simulink model "pe_electric_engine_dyno"  (R2017b)
settings: Solver=FixedStepDiscrete  StartTime=0.0  StopTime=0.8  FixedStep=Ts  RelTol=1e-3  EnableMultiTasking=on
PreLoadFcn:
  | pe_electric_engine_dyno_data;
values from neighbouring files (symbols this model uses):
  ce = 25    [pe_electric_engine_dyno_data.m]
  fn = 60    [pe_electric_engine_dyno_data.m]
  Ibase = Pn/(1.5*Vbase)    [pe_electric_engine_dyno_data.m]
  Ld = 0.00024368    [pe_electric_engine_dyno_data.m]
  Lm = 2.717    [pe_electric_engine_dyno_data.m]
  Lq = 0.00029758    [pe_electric_engine_dyno_data.m]
  p = 8    [pe_electric_engine_dyno_data.m]
  p2 = 2    [pe_electric_engine_dyno_data.m]
  psim = 0.04366    [pe_electric_engine_dyno_data.m]
  Ts = 5e-6    (= 5e-06)    [init_model_Ffwd.m]    (also in pe_electric_engine_dyno_data.m = 1e-05)
  Tsc = 1/(fsw2*5)    (= 0.0001)    [pe_electric_engine_dyno_data.m]
  Xls = Lls*Zbase    [pe_electric_engine_dyno_data.m]
undefined symbols (not defined in the file or in its folder): pe, sigbuilder_block, VDC_VECT
libraries: nesl_utility x22, fl_lib x15, pe_lib x12, peTransforms x2, peAsmFieldOrientedControl x1, peGeneralControl x1, pePmsmCurrentController x1, simulink x1, pePmsmCurrentReferenceGen x1, pePmsmTorqueEstimator x1, pePwmGeneratorTwoLevel x1
Description:
  | Electric Engine Dyno
  | 
  | This example shows how to model an electric vehicle dynamometer test.
  | The test environment contains an asynchronous machine (ASM) and an
  | interior permanent magnet synchronous machine (IPMSM) connected back-
  | to-back through a mechanical shaft. Both machines are fed by high-
  | voltage batteries through controlled three-phase converters. The 164 kW
  | ASM produces the load torque. The 35 kW IPMSM is the electric machine
  | under test. The Control Machine Under Test (IPMSM) subsystem controls the
  | torque of the IPMSM. The controller includes a multi-rate PI-based
  | control structure. The rate of the open-loop torque control is slower
  | than the rate of the closed-loop current control. The task scheduling
  | for the controller is implemented as a Stateflow(TM) state machine. The
  | Control Load Machine (ASM) subsystem uses a single rate to control the
  | speed of the ASM. The Visualization subsystem contains scopes that
  | allow you to see the simulation results.
settings Model: Creator=The MathWorks, Inc.  LastModifiedBy=The MathWorks, Inc.
settings OptimizationCC: LifeSpan=inf
settings DebuggingCC: UnderspecifiedInitializationDetection=Classic  MergeDetectMultiDrivingBlocksExec=none  SFUnexpectedBacktrackingDiag=warning  SFNoUnconditionalDefaultTransitionDiag=warning  SFExecutionAtInitializationDiag=none
settings CodeAppCC: StateflowObjectComments=on
settings GRTTargetCC: TargetLangStandard=C89/C90 (ANSI)  GeneratePreprocessorConditionals=Disable all
settings ConfigComp: CovMetricSettings=dw  CovHtmlReporting=on  CovSaveCumulativeToWorkspaceVar=on  CovSaveSingleToWorkspaceVar=on  CovExternalEMLEnable=off
settings SimscapeCC: SimscapeLogType=all  SimscapeLogSimulationStatistics=on  SimscapeLogName=simlog_pe_electric_engine_dyno  SimscapeLogLimitData=off

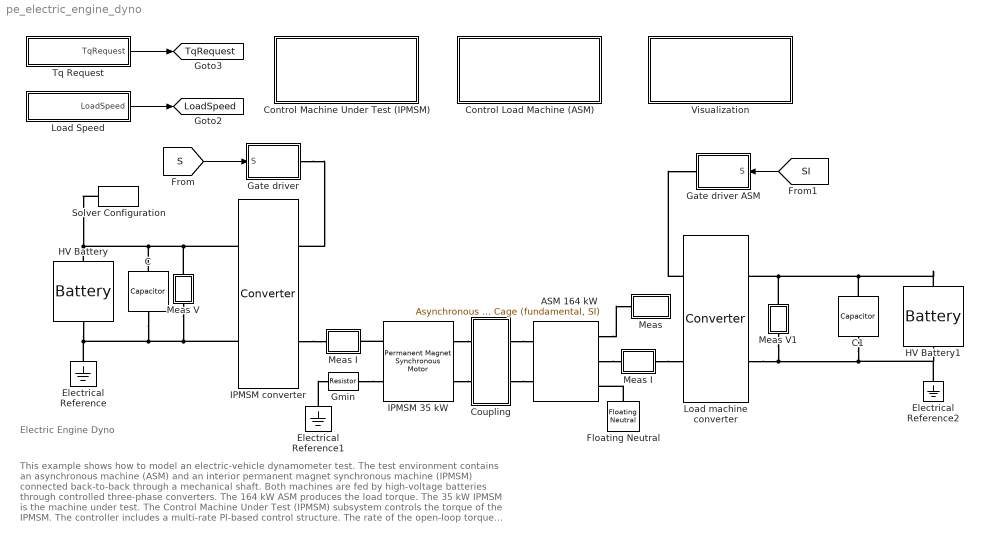
== system pe_electric_engine_dyno ==
  note: This example shows how to model an electric-vehicle dynamometer test. The test environment contains an asynchronous machine (ASM) and an interior permanent magnet synchronous machine (IPMSM) connected back-to-back through a mechanical shaft. Both machines are fed by high-voltage batteries through controlled three-phase converters. The 164 kW ASM produces the load torque. The 35 kW IPMSM is the machine under test. The Control Machine Under Test (IPMSM) subsystem controls the torque of the IPMSM. The controller includes a multi-rate PI-based control structure. The rate of the open-loop torque control is slower than the rate of the closed-loop current control. The task scheduling for the controller is implemented as a Stateflow(TM) state machine. The Control Load Machine (ASM) subsystem uses a single rate to control the speed of the ASM. The Visualization subsystem contains scopes that allow you to see the simulation results.
      | Edit associated parameterization script.
      | Explore simulation results using sscexplore .
      | Learn more about this example.
  note: Electric Engine Dyno
  ASM 164 kW : pe_lib/Machines/Asynchronous Machine (Squirrel Cage)/Asynchronous Machine Squirrel Cage (fundamental, SI)  SRated=Pn V*A  VRated=Vn V  FRated=fn Hz  nPolePairs=p2  Rs=Rss Ohm  Xls=Xls Ohm  Rrd=Rrr Ohm  Xlrd=Xlr Ohm  Xm=Xm Ohm  X0=Xls Ohm  angular_position0=0 deg  psids0=0 Wb  psiqs0=0 Wb  psi0s0=0 Wb  psidr0=0 Wb  psiqr0=0 Wb  connection_option=int32(pe.Connection.delta)
      settings: SourceProductName=Simscape Power Systems  SourceProductBaseCode=PS
  C : fl_lib/Electrical/Electrical Elements/Capacitor  c=Cdc F  r=1e-6 Ohm  g=0 1/Ohm  i_specify=off  i_priority=None  i=0 A  i_nominal_specify=off  i_nominal_unit=A  i_nominal_value=1  v_specify=off  v_priority=None  v=0 V  v_nominal_specify=off  v_nominal_unit=V  v_nominal_value=1  vc_specify=off  vc_priority=High  vc=0 V  vc_nominal_specify=off  vc_nominal_unit=V  vc_nominal_value=1
      settings: SourceProductName=Foundation Library
  C1 : fl_lib/Electrical/Electrical Elements/Capacitor  c=Cdc F  r=1e-6 Ohm  g=0 1/Ohm  i_specify=off  i_priority=None  i=0 A  i_nominal_specify=off  i_nominal_unit=A  i_nominal_value=1  v_specify=off  v_priority=None  v=0 V  v_nominal_specify=off  v_nominal_unit=V  v_nominal_value=1  vc_specify=off  vc_priority=High  vc=0 V  vc_nominal_specify=off  vc_nominal_unit=V  vc_nominal_value=1
      settings: SourceProductName=Foundation Library
  Control Load Machine (ASM) : Subsystem
  Control Machine Under Test (IPMSM) : Subsystem
  Coupling : Subsystem
  Electrical Reference : fl_lib/Electrical/Electrical Elements/Electrical Reference
      settings: SourceProductName=Foundation Library
  Electrical Reference1 : fl_lib/Electrical/Electrical Elements/Electrical Reference
      settings: SourceProductName=Foundation Library
  Electrical Reference2 : fl_lib/Electrical/Electrical Elements/Electrical Reference
      settings: SourceProductName=Foundation Library
  Floating Neutral : pe_lib/Connections/Floating Neutral
      settings: SourceProductName=Simscape Power Systems  SourceProductBaseCode=PS
  Gate driver : Subsystem
  Gate driver ASM : Subsystem
  Gmin : fl_lib/Electrical/Electrical Elements/Resistor  R=1e9 Ohm  i_specify=off  i_priority=High  i=0 A  i_nominal_specify=off  i_nominal_unit=A  i_nominal_value=1  v_specify=off  v_priority=High  v=0 V  v_nominal_specify=off  v_nominal_unit=V  v_nominal_value=1
      settings: SourceProductName=Foundation Library
  HV Battery : pe_lib/Sources/Battery  Vnom=Vnom V  R1=0.001 Ohm  prm_AH=2  AH=10000 hr*A  V1=V1 V  AH1=3000 hr*A  prm_R2=1  R2=2000 Ohm  prm_fade=1  N_fade=100  AH_fade=45 hr*A  R1_fade=2.02 Ohm  V1_fade=10.35 V  i_specify=off  i_priority=None  i=0 A  i_nominal_specify=off  i_nominal_unit=A  i_nominal_value=1  v_specify=off  v_priority=None  v=0 V  v_nominal_specify=off  v_nominal_unit=V  v_nominal_value=1  charge_specify=on  charge_priority=High  charge=8000 hr*A  charge_nominal_specify=off  charge_nominal_unit=hr*A  charge_nominal_value=1  num_cycles_specify=off  num_cycles_priority=High  num_cycles=0  num_cycles_nominal_specify=off  num_cycles_nominal_unit=1  num_cycles_nominal_value=1  thermal_mass=30000 J/K  Tmeas=298.15 K  Vnom_T2=12 V  R1_T2=2.2 Ohm  V1_T2=11.4 V  R2_T2=2200 Ohm  Tmeas2=273.15 K  temperature_specify=off  temperature_priority=High  temperature=298.15 K  temperature_nominal_specify=off  temperature_nominal_unit=K  temperature_nominal_value=1
      settings: SourceProductName=Simscape Power Systems  SourceProductBaseCode=PS
  HV Battery1 : pe_lib/Sources/Battery  Vnom=775 V  R1=0.001 Ohm  prm_AH=2  AH=25000 hr*A  V1=750 V  AH1=20000 hr*A  prm_R2=1  R2=2000 Ohm  prm_fade=1  N_fade=100  AH_fade=45 hr*A  R1_fade=2.02 Ohm  V1_fade=10.35 V  i_specify=off  i_priority=None  i=0 A  i_nominal_specify=off  i_nominal_unit=A  i_nominal_value=1  v_specify=off  v_priority=None  v=0 V  v_nominal_specify=off  v_nominal_unit=V  v_nominal_value=1  charge_specify=on  charge_priority=High  charge=20000 hr*A  charge_nominal_specify=off  charge_nominal_unit=hr*A  charge_nominal_value=1  num_cycles_specify=off  num_cycles_priority=High  num_cycles=0  num_cycles_nominal_specify=off  num_cycles_nominal_unit=1  num_cycles_nominal_value=1  thermal_mass=30000 J/K  Tmeas=298.15 K  Vnom_T2=12 V  R1_T2=2.2 Ohm  V1_T2=11.4 V  R2_T2=2200 Ohm  Tmeas2=273.15 K  temperature_specify=off  temperature_priority=High  temperature=298.15 K  temperature_nominal_specify=off  temperature_nominal_unit=K  temperature_nominal_value=1
      settings: SourceProductName=Simscape Power Systems  SourceProductBaseCode=PS
  IPMSM 35 kW : pe_lib/Machines/Permanent Magnet Rotor/Permanent Magnet Synchronous Motor  nPolePairs=p  pmflux_param=1  pm_flux_linkage=psim Wb  torque_constant=0.18 N*m/A  back_emf_constant=0.18 V/(rad/s)  stator_param=1  Ld=Ld H  Lq=Lq H  L0=L0 H  Ls=0.0002 H  Lm=0.00002 H  Ms=0.00002 H  Rs=Rs Ohm  initial_currents=[0, 0, 0] A  axes_param=1  angular_position0=0 rad  rotor_offset=- pi / 2 rad  shift_3ph=[nan, nan, nan] rad  sqrt2OverSqrt3=nan  oneOverSqrt2=nan  twoPiOver3=nan  Lmin=1e-9 H
      settings: SourceProductName=Simscape Power Systems  SourceProductBaseCode=PS
  IPMSM converter : pe_lib/Semiconductors/Converter  device_type=3  Vf=0.8 V  Ron=0.001 Ohm  Rds=0.001 Ohm  Goff=1e-5 1/Ohm  Vth=0.5 V  Vgt=1 V  Vgt_off=-1 V  Ih=1 A  diode_param=2  diode_Vf=0.8 V  diode_Ron=0.001 Ohm  diode_Goff=1e-5 1/Ohm  diode_C=50 nF  diode_iRM=-235 A  diode_iF=300 A  diode_idot=-50 A/us  diode_trr_param=1  diode_trr_factor=3  diode_trr=15 us  diode_Qrr=1.5e+3 s*uA  snubber_type=0  Rs=0.1 Ohm  Cs=1e-7 F
      settings: SourceProductName=Simscape Power Systems  SourceProductBaseCode=PS
  Load Speed : Subsystem  Tag=STV Subsys  LoadFcn=sigbuilder_block('load');  StartFcn=sigbuilder_block('start');  StopFcn=sigbuilder_block('stop');  ClipboardFcn=sigbuilder_block('clipboard');  mask(Sigbuilder block){tuvar=[0:10]}
      mask help: Simulink:masks:SigbuilderBlock_MD
      mask init:
      | if ~strcmp(get_param(bdroot(gcbh),'SimulationStatus'),'stopped') tuvar = sigbuilder_block('maskInit'); end
      settings: CopyFcn=sigbuilder_block('copy');  DeleteFcn=sigbuilder_block('delete');  ModelCloseFcn=sigbuilder_block('modelClose');  PreSaveFcn=sigbuilder_block('preSave');  PauseFcn=sigbuilder_block('pause');  ContinueFcn=sigbuilder_block('continue');  NameChangeFcn=sigbuilder_block('namechange');  OpenFcn=sigbuilder_block('open',[324 245.25 633.75 283.5 ]);  CloseFcn=sigbuilder_block('close');
      mask Display: plot(0, 0, 100, 100,[2, 2, 32, 32, 2], [68, 8, 8, 68, 68],[32, 2], [38, 38], [32, 19, 2],[53, 60, 44], [32, 17, 17, 2],[16, 16, 31, 31]);txt = getActiveGroup(gcbh);text(2, 100, txt,'verticalAlignment', 'top');
  Load machine converter : pe_lib/Semiconductors/Converter  device_type=3  Vf=0.8 V  Ron=0.001 Ohm  Rds=0.001 Ohm  Goff=1e-5 1/Ohm  Vth=0.5 V  Vgt=1 V  Vgt_off=-1 V  Ih=1 A  diode_param=2  diode_Vf=0.8 V  diode_Ron=0.001 Ohm  diode_Goff=1e-5 1/Ohm  diode_C=50 nF  diode_iRM=-235 A  diode_iF=300 A  diode_idot=-50 A/us  diode_trr_param=1  diode_trr_factor=3  diode_trr=15 us  diode_Qrr=1.5e+3 s*uA  snubber_type=0  Rs=0.1 Ohm  Cs=1e-7 F
      settings: SourceProductName=Simscape Power Systems  SourceProductBaseCode=PS
  Meas : Subsystem
  Meas I : Subsystem
  "Meas I " : Subsystem
  Meas V : Subsystem
  Meas V1 : Subsystem
  Solver Configuration : nesl_utility/Solver Configuration  PhysicalDomain=network_engine_domain  SubClassName=solver  LeftPortType=input  RightPortType=generic  Accelerate=off  Tones=[]  Harmonics=[]  SimulateNoise=off  Profile=off  UseLocalSampling=off  EnableSwitchedLinearOptims=on  FrequencyDomain=off  UseCCode=off  RelTol=0.001  AbsTol=1e-06  MinStep=1e-09  ToWorkspace=off  RevertToSquareIcSolve=off  NumHomotopyIterations=100  PhasorMode=off  PhasorModeNumHarmonics=1  DoDC=off  ResidualTolerance=1e-9  UseLocalSolver=on  LocalSolverChoice=NE_BACKWARD_EULER_ADVANCER  LocalSolverSampleTime=Ts  DoFixedCost=on  MaxNonlinIter=4  MaxModeIter=2  LinearAlgebra=Sparse  DelaysMemoryBudget=1024  AutomaticFiltering=on  FilteringTimeConstant=0.001
  Tq Request : Subsystem  Tag=STV Subsys  LoadFcn=sigbuilder_block('load');  StartFcn=sigbuilder_block('start');  StopFcn=sigbuilder_block('stop');  ClipboardFcn=sigbuilder_block('clipboard');  mask(Sigbuilder block){tuvar=[0:10]}
      mask help: Simulink:masks:SigbuilderBlock_MD
      mask init:
      | if ~strcmp(get_param(bdroot(gcbh),'SimulationStatus'),'stopped') tuvar = sigbuilder_block('maskInit'); end
      settings: CopyFcn=sigbuilder_block('copy');  DeleteFcn=sigbuilder_block('delete');  ModelCloseFcn=sigbuilder_block('modelClose');  PreSaveFcn=sigbuilder_block('preSave');  PauseFcn=sigbuilder_block('pause');  ContinueFcn=sigbuilder_block('continue');  NameChangeFcn=sigbuilder_block('namechange');  OpenFcn=sigbuilder_block('open',[1556.25 287.25 486.75 260.25 ]);  CloseFcn=sigbuilder_block('close');
      mask Display: plot(0, 0, 100, 100,[2, 2, 32, 32, 2], [68, 8, 8, 68, 68],[32, 2], [38, 38], [32, 19, 2],[53, 60, 44], [32, 17, 17, 2],[16, 16, 31, 31]);txt = getActiveGroup(gcbh);text(2, 100, txt,'verticalAlignment', 'top');
  Visualization : Subsystem
  tag scope: LoadSpeed=global, TqRequest=global
  wires:
  [S] -> Gate driver/1(S)
  [SI] -> Gate driver ASM/1(S)
  Tq Request/1(TqRequest) -> [TqRequest]
  Load Speed/1(LoadSpeed) -> [LoadSpeed]
  connections:
  IPMSM converter/RConn2 -- Meas V/RConn1 -- HV Battery/RConn1 -- Electrical Reference/LConn1 -- C/RConn1
  IPMSM converter/RConn1 -- Meas V/LConn1 -- HV Battery/LConn1 -- Solver Configuration/RConn1 -- C/LConn1
  Electrical Reference1/LConn1 -- Gmin/LConn1
  Gate driver/RConn1 -- IPMSM converter/LConn1
  Floating Neutral/LConn1 -- ASM 164 kW/RConn3
  HV Battery1/LConn1 -- C1/LConn1 -- Load machine converter/RConn1 -- Meas V1/LConn1
  Load machine converter/RConn2 -- Meas V1/RConn1 -- Electrical Reference2/LConn1 -- HV Battery1/RConn1 -- C1/RConn1
  IPMSM 35 kW/RConn2 -- Coupling/LConn2
  Coupling/RConn2 -- ASM 164 kW/LConn2
  IPMSM 35 kW/RConn1 -- Coupling/LConn1
  IPMSM converter/LConn2 -- Meas I/LConn1
  IPMSM 35 kW/LConn1 -- Meas I/RConn1
  Coupling/RConn1 -- ASM 164 kW/LConn1
  Gmin/RConn1 -- IPMSM 35 kW/LConn2
  ASM 164 kW/RConn2 -- "Meas I "/RConn1
  "Meas I "/LConn1 -- Load machine converter/LConn2
  ASM 164 kW/RConn1 -- Meas/LConn1
  Load machine converter/LConn1 -- Gate driver ASM/RConn1

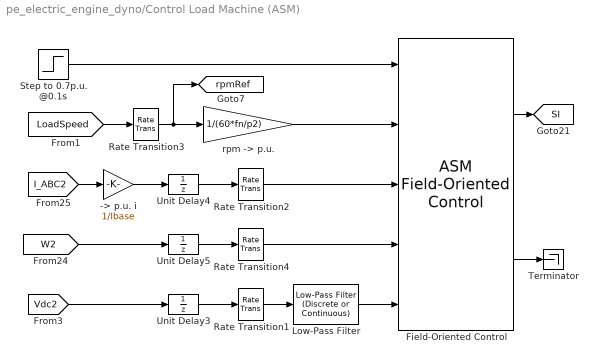
== system pe_electric_engine_dyno/Control Load Machine (ASM) ==
  -> p.u. i : Gain  Gain=1/Ibase
  Field-Oriented Control : peAsmFieldOrientedControl/ASM Field-Oriented Control  Vn=Vn  fn=fn  Rr=Rr  Llr=Llr  Lm=Lm  Tc=1e-4  Vdc_on=400  Ts=Ts  Tsc=Tsc  Kp_imr=Kp_imr  Ki_imr=Ki_imr  Kaw_imr=1000  Kp_wr=Kp_wr  Ki_wr=Ki_wr  Kaw_wr=1000  id_max=2  iq_max=2  AxisAlignment=Q-axis  Kp_id=Kp_ids  Ki_id=Ki_ids  Kaw_id=1000  Kp_iq=Kp_iqs  Ki_iq=Ki_iqs  Kaw_iq=1000  AxisPrio=D-Q equivalence  CPWMMode=SPWM: sinusoidal PWM  fsw=fsw2
      settings: SamplingMode=Natural
  Low-Pass Filter : peGeneralControl/Low-Pass Filter (Discrete or Continuous)  K=1  T=1e-3  B=inf  A=-inf  Ts=Tsc
  Rate Transition{1..4} (4 alike) : RateTransition  OutPortSampleTime=Tsc
  Step to 0.7p.u. @0.1s : Step  Time=0.1  After=0.7*1/Lm  SampleTime=Tsc
  Terminator : Terminator
  Unit Delay3 : UnitDelay  SampleTime=Ts
  Unit Delay4 : UnitDelay  SampleTime=Ts
  Unit Delay5 : UnitDelay  SampleTime=Ts
  "rpm -> p.u." : Gain  Gain=1/(60*fn/p2)
  tag scope: SI=global, rpmRef=global
  wires:
  [LoadSpeed] -> Rate Transition3/1
  Field-Oriented Control/1 -> [SI]
  Unit Delay5/1 -> Rate Transition4/1
  [Vdc2] -> Unit Delay3/1
  Rate Transition2/1 -> Field-Oriented Control/3
  Low-Pass Filter/1 -> Field-Oriented Control/5
  Rate Transition1/1 -> Low-Pass Filter/1
  [W2] -> Unit Delay5/1
  Rate Transition4/1 -> Field-Oriented Control/4
  Unit Delay4/1 -> Rate Transition2/1
  Unit Delay3/1 -> Rate Transition1/1
  [I_ABC2] -> -> p.u. i/1
  -> p.u. i/1 -> Unit Delay4/1
  Rate Transition3/1 -> [rpmRef], "rpm -> p.u."/1
  Step to 0.7p.u. @0.1s/1 -> Field-Oriented Control/1
  "rpm -> p.u."/1 -> Field-Oriented Control/2
  Field-Oriented Control/2 -> Terminator/1

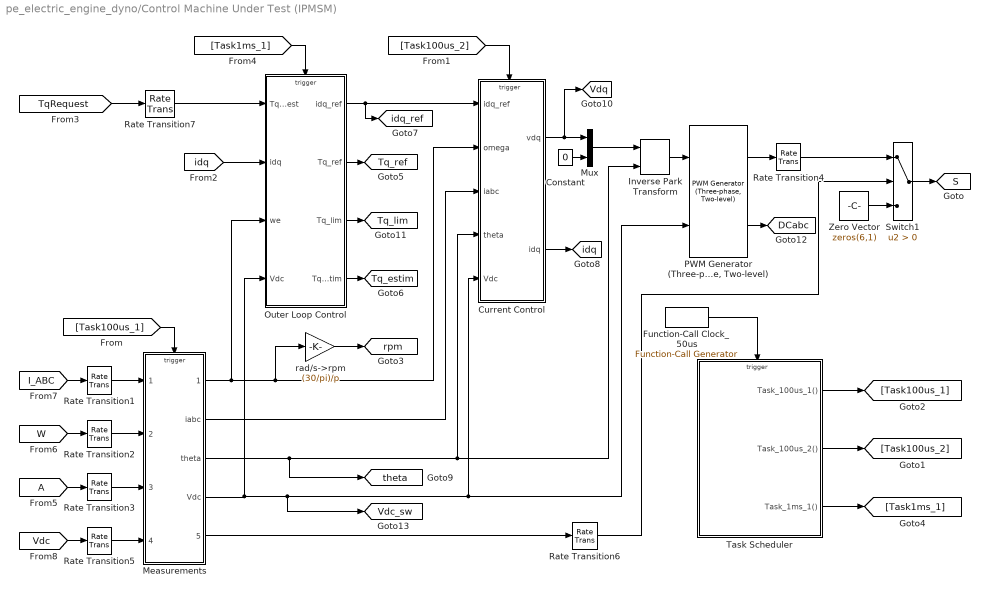
== system pe_electric_engine_dyno/Control Machine Under Test (IPMSM) ==
  Constant : Constant  Value=0  SampleTime=-1
  Current Control : Subsystem
  Function-Call Clock_50us : simulink/Ports & Subsystems/Function-Call Generator  sample_time=5e-5  numberOfIterations=1
  Inverse Park Transform : peTransforms/Inverse Park Transform  AxisAlignment=Q-axis  PowerInvariant=off
  Measurements : Subsystem
  Mux : Mux  Inputs=2
  Outer Loop Control : Subsystem
  "PWM Generator (Three-phase, Two-level)" : pePwmGeneratorTwoLevel/PWM Generator (Three-phase, Two-level)  OverrideUsingVariant=NaturalMode  PWMMode=Continuous PWM (CPWM)  CPWMMode=SVM: space vector modulation  DPWMMode=60 DPWM: 60 degree discontinuous PWM  fsw=fsw  Ts=Ts
      settings: SamplingMode=Natural
  Rate Transition{1..7} (7 alike) : RateTransition
  Switch1 : Switch  Criteria=u2 > Threshold
  Task Scheduler : Stateflow chart  TreatAsAtomicUnit=on
  Zero Vector : Constant  Value=zeros(6,1)  SampleTime=-1
  rad/s->rpm : Gain  Gain=(30/pi)/p
  tag scope: DCabc=global, S=global, Tq_estim=global, Tq_lim=global, Tq_ref=global, Vdc_sw=global, Vdq=global, idq=global, idq_ref=global, rpm=global, theta=global
  wires:
  Current Control/1(vdq) -> Mux/1, [Vdq]
  Measurements/2(iabc) -> Current Control/3(iabc)
  Measurements/3(theta) -> [theta], Inverse Park Transform/2, Current Control/4(theta)
  "PWM Generator (Three-phase, Two-level)"/1 -> Rate Transition4/1
  Inverse Park Transform/1 -> "PWM Generator (Three-phase, Two-level)"/1
  [I_ABC] -> Rate Transition1/1
  [W] -> Rate Transition2/1
  [A] -> Rate Transition3/1
  [Vdc] -> Rate Transition5/1
  Outer Loop Control/1(idq_ref) -> Current Control/1(idq_ref), [idq_ref]
  "PWM Generator (Three-phase, Two-level)"/2 -> [DCabc]
  Rate Transition1/1 -> Measurements/1(iabc_m)
  Rate Transition2/1 -> Measurements/2(omega_m)
  Rate Transition3/1 -> Measurements/3(theta_m)
  Rate Transition5/1 -> Measurements/4(Vdc_m)
  Function-Call Clock_50us/1 -> Task Scheduler/Trigger
  Task Scheduler/3(Task_1ms_1()) -> [Task1ms_1]
  Task Scheduler/2(Task_100us_2()) -> [Task100us_2]
  Task Scheduler/1(Task_100us_1()) -> [Task100us_1]
  Outer Loop Control/2(Tq_ref) -> [Tq_ref]
  Measurements/1(omega) -> Current Control/2(omega), rad/s->rpm/1, Outer Loop Control/3(we)
  rad/s->rpm/1 -> [rpm]
  Outer Loop Control/3(Tq_lim) -> [Tq_lim]
  Rate Transition7/1 -> Outer Loop Control/1(TqRequest)
  [TqRequest] -> Rate Transition7/1
  Outer Loop Control/4(Tq_estim) -> [Tq_estim]
  [idq] -> Outer Loop Control/2(idq)
  Measurements/4(Vdc) -> [Vdc_sw], "PWM Generator (Three-phase, Two-level)"/2, Current Control/5(Vdc), Outer Loop Control/4(Vdc)
  Rate Transition4/1 -> Switch1/1
  Switch1/1 -> [S]
  Measurements/5(PwmON) -> Rate Transition6/1
  Zero Vector/1 -> Switch1/3
  Rate Transition6/1 -> Switch1/2
  [Task100us_2] -> Current Control/Trigger
  [Task1ms_1] -> Outer Loop Control/Trigger
  [Task100us_1] -> Measurements/Trigger
  Current Control/2(idq) -> [idq]
  Constant/1 -> Mux/2
  Mux/1 -> Inverse Park Transform/1

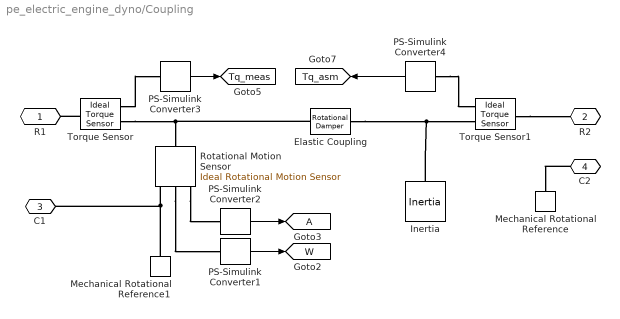
== system pe_electric_engine_dyno/Coupling ==
  Elastic Coupling : fl_lib/Mechanical/Rotational Elements/Rotational Damper  D=ce N*m/(rad/s)  w_specify=off  w_priority=None  w=0 rad/s  w_nominal_specify=off  w_nominal_unit=rad/s  w_nominal_value=1  t_specify=off  t_priority=None  t=0 N*m  t_nominal_specify=off  t_nominal_unit=N*m  t_nominal_value=1
      settings: LogSimulationData=on
  Inertia : fl_lib/Mechanical/Rotational Elements/Inertia  inertia=Jm kg*m^2  w_specify=off  w_priority=High  w=0 rad/s  w_nominal_specify=off  w_nominal_unit=rad/s  w_nominal_value=1  t_specify=off  t_priority=None  t=0 N*m  t_nominal_specify=off  t_nominal_unit=N*m  t_nominal_value=1
      settings: SourceProductName=Foundation Library
  Mechanical Rotational Reference : fl_lib/Mechanical/Rotational Elements/Mechanical Rotational Reference
      settings: SourceProductName=Foundation Library
  Mechanical Rotational Reference1 : fl_lib/Mechanical/Rotational Elements/Mechanical Rotational Reference
      settings: SourceProductName=Foundation Library
  PS-Simulink Converter1 : nesl_utility/PS-Simulink Converter  PhysicalDomain=network_engine_domain  SubClassName=ps_output  LeftPortType=input  RightPortType=output  PseudoPeriodic=off  Frequencies=[]  Unit=rad/s  AffineConversion=off
  PS-Simulink Converter2 : nesl_utility/PS-Simulink Converter  PhysicalDomain=network_engine_domain  SubClassName=ps_output  LeftPortType=input  RightPortType=output  PseudoPeriodic=off  Frequencies=[]  Unit=rad  AffineConversion=off
  PS-Simulink Converter3 : nesl_utility/PS-Simulink Converter  PhysicalDomain=network_engine_domain  SubClassName=ps_output  LeftPortType=input  RightPortType=output  PseudoPeriodic=off  Frequencies=[]  Unit=N*m  AffineConversion=off
  PS-Simulink Converter4 : nesl_utility/PS-Simulink Converter  PhysicalDomain=network_engine_domain  SubClassName=ps_output  LeftPortType=input  RightPortType=output  PseudoPeriodic=off  Frequencies=[]  Unit=N*m  AffineConversion=off
  Rotational Motion Sensor : fl_lib/Mechanical/Mechanical Sensors/Ideal Rotational Motion Sensor  offset=0 deg
      settings: SourceProductName=Foundation Library
  Torque Sensor : fl_lib/Mechanical/Mechanical Sensors/Ideal Torque Sensor
      settings: SourceProductName=Foundation Library
  Torque Sensor1 : fl_lib/Mechanical/Mechanical Sensors/Ideal Torque Sensor
      settings: SourceProductName=Foundation Library
  R1 : PMIOPort  Port=1  Side=Left
  R2 : PMIOPort  Port=2  Side=Right
  C1 : PMIOPort  Port=3  Side=Left
  C2 : PMIOPort  Port=4  Side=Right
  tag scope: A=global, Tq_asm=global, Tq_meas=global, W=global
  wires:
  PS-Simulink Converter2/1 -> [A]
  PS-Simulink Converter1/1 -> [W]
  PS-Simulink Converter3/1 -> [Tq_meas]
  PS-Simulink Converter4/1 -> [Tq_asm]
  connections:
  Rotational Motion Sensor/RConn2 -- PS-Simulink Converter1/LConn1
  Mechanical Rotational Reference1/LConn1 -- C1/RConn1 -- Rotational Motion Sensor/RConn1
  Rotational Motion Sensor/RConn3 -- PS-Simulink Converter2/LConn1
  C2/RConn1 -- Mechanical Rotational Reference/LConn1
  Torque Sensor/RConn1 -- Elastic Coupling/LConn1 -- Rotational Motion Sensor/LConn1
  Torque Sensor/LConn1 -- R1/RConn1
  Torque Sensor/RConn2 -- PS-Simulink Converter3/LConn1
  Torque Sensor1/LConn1 -- R2/RConn1
  PS-Simulink Converter4/LConn1 -- Torque Sensor1/RConn2
  Inertia/LConn1 -- Torque Sensor1/RConn1 -- Elastic Coupling/RConn1

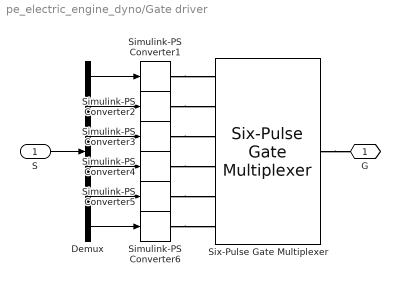
== system pe_electric_engine_dyno/Gate driver ==
  S : Inport
  Demux : Demux  Outputs=6
  Simulink-PS Converter{1..6} (6 alike) : nesl_utility/Simulink-PS Converter  PhysicalDomain=network_engine_domain  SubClassName=ps_input  LeftPortType=input  RightPortType=output  PseudoPeriodic=off  Frequencies=[]  NoiseDistribution=none  NoiseParameters=[]  Unit=1  AffineConversion=off  FilteringAndDerivatives=zero  SimscapeFilterOrder=1  InputFilterTimeConstant=0.001  UdotUserProvided=1
  Six-Pulse Gate Multiplexer : pe_lib/Semiconductors/Six-Pulse Gate Multiplexer  R=0 Ohm
      settings: SourceProductName=Simscape Power Systems  SourceProductBaseCode=PS
  G : PMIOPort  Port=1  Side=Right
  wires:
  Demux/1 -> Simulink-PS Converter1/1
  S/1 -> Demux/1
  Demux/4 -> Simulink-PS Converter4/1
  Demux/2 -> Simulink-PS Converter2/1
  Demux/3 -> Simulink-PS Converter3/1
  Demux/5 -> Simulink-PS Converter5/1
  Demux/6 -> Simulink-PS Converter6/1
  connections:
  Six-Pulse Gate Multiplexer/RConn1 -- G/RConn1
  Simulink-PS Converter1/RConn1 -- Six-Pulse Gate Multiplexer/LConn1
  Simulink-PS Converter3/RConn1 -- Six-Pulse Gate Multiplexer/LConn3
  Simulink-PS Converter5/RConn1 -- Six-Pulse Gate Multiplexer/LConn5
  Simulink-PS Converter6/RConn1 -- Six-Pulse Gate Multiplexer/LConn6
  Simulink-PS Converter4/RConn1 -- Six-Pulse Gate Multiplexer/LConn4
  Simulink-PS Converter2/RConn1 -- Six-Pulse Gate Multiplexer/LConn2

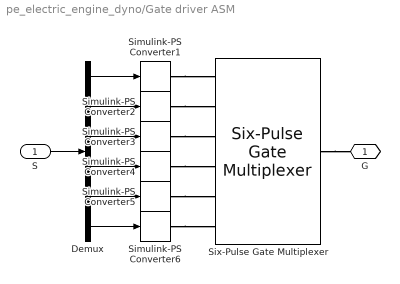
== system pe_electric_engine_dyno/Gate driver ASM ==
  S : Inport
  Demux : Demux  Outputs=6
  Simulink-PS Converter{1..6} (6 alike) : nesl_utility/Simulink-PS Converter  PhysicalDomain=network_engine_domain  SubClassName=ps_input  LeftPortType=input  RightPortType=output  PseudoPeriodic=off  Frequencies=[]  NoiseDistribution=none  NoiseParameters=[]  Unit=1  AffineConversion=off  FilteringAndDerivatives=zero  SimscapeFilterOrder=1  InputFilterTimeConstant=0.001  UdotUserProvided=1
  Six-Pulse Gate Multiplexer : pe_lib/Semiconductors/Six-Pulse Gate Multiplexer  R=0 Ohm
      settings: SourceProductName=Simscape Power Systems  SourceProductBaseCode=PS
  G : PMIOPort  Port=1  Side=Right
  wires:
  Demux/6 -> Simulink-PS Converter6/1
  Demux/5 -> Simulink-PS Converter5/1
  Demux/3 -> Simulink-PS Converter3/1
  Demux/2 -> Simulink-PS Converter2/1
  Demux/4 -> Simulink-PS Converter4/1
  S/1 -> Demux/1
  Demux/1 -> Simulink-PS Converter1/1
  connections:
  Simulink-PS Converter2/RConn1 -- Six-Pulse Gate Multiplexer/LConn2
  Simulink-PS Converter4/RConn1 -- Six-Pulse Gate Multiplexer/LConn4
  Simulink-PS Converter6/RConn1 -- Six-Pulse Gate Multiplexer/LConn6
  Simulink-PS Converter5/RConn1 -- Six-Pulse Gate Multiplexer/LConn5
  Simulink-PS Converter3/RConn1 -- Six-Pulse Gate Multiplexer/LConn3
  Simulink-PS Converter1/RConn1 -- Six-Pulse Gate Multiplexer/LConn1
  Six-Pulse Gate Multiplexer/RConn1 -- G/RConn1

== system pe_electric_engine_dyno/Load Speed ==
  Demux : Demux  Tag=STV Demux  Outputs=1
  FromWs : FromWorkspace  Tag=STV FromWs  VariableName=tuvar  SampleTime=0
      SigBuilderData=|
      | common.afterFinalStr = 'Extrapolate'
      | common.sampleTime = 0
      | dataSet.timeRange = [0 0.8]
      | dataSet.name = 'Group 1'
      | sbobj.Groups.Name = 'Group 1'
      | sbobj.Groups.Signals.Name = 'LoadSpeed'
      | sbobj.Groups.Signals.XData = [0 0.1 0.2 0.6 0.6 0.644 0.8]
      | sbobj.Groups.Signals.YData = [0 0 1000 1000 1010 2350 2350]
      | sbobj.Groups.TimeRange = [0 0.8]
  LoadSpeed : Outport  Tag=STV Outport
  wires:
  Demux/1 -> LoadSpeed/1
  FromWs/1 -> Demux/1

== system pe_electric_engine_dyno/Meas ==
  PS-Simulink Converter5 : nesl_utility/PS-Simulink Converter  PhysicalDomain=network_engine_domain  SubClassName=ps_output  LeftPortType=input  RightPortType=output  PseudoPeriodic=off  Frequencies=[]  Unit=1  AffineConversion=off
  Rotor speed : pe_lib/Machines/Asynchronous Machine Measurement  output_idx=2
      settings: SourceProductName=Simscape Power Systems  SourceProductBaseCode=PS
  pu : PMIOPort  Port=1  Side=Left
  tag scope: W2=global
  wires:
  PS-Simulink Converter5/1 -> [W2]
  connections:
  Rotor speed/LConn1 -- pu/RConn1
  Rotor speed/RConn1 -- PS-Simulink Converter5/LConn1

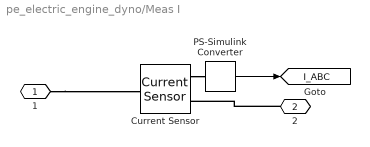
== system pe_electric_engine_dyno/Meas I ==
  Current Sensor : pe_lib/Sensors/Current Sensor
      settings: SourceProductName=Simscape Power Systems  SourceProductBaseCode=PS
  PS-Simulink Converter : nesl_utility/PS-Simulink Converter  PhysicalDomain=network_engine_domain  SubClassName=ps_output  LeftPortType=input  RightPortType=output  PseudoPeriodic=off  Frequencies=[]  Unit=A  AffineConversion=off
  1 : PMIOPort  Port=1  Side=Left
  2 : PMIOPort  Port=2  Side=Right
  tag scope: I_ABC=global
  wires:
  PS-Simulink Converter/1 -> [I_ABC]
  connections:
  1/RConn1 -- Current Sensor/LConn1
  2/RConn1 -- Current Sensor/RConn2
  Current Sensor/RConn1 -- PS-Simulink Converter/LConn1

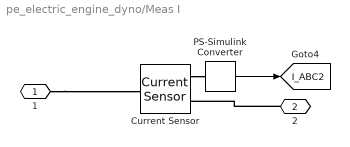
== system pe_electric_engine_dyno/Meas I  ==
  Current Sensor : pe_lib/Sensors/Current Sensor
      settings: SourceProductName=Simscape Power Systems  SourceProductBaseCode=PS
  PS-Simulink Converter : nesl_utility/PS-Simulink Converter  PhysicalDomain=network_engine_domain  SubClassName=ps_output  LeftPortType=input  RightPortType=output  PseudoPeriodic=off  Frequencies=[]  Unit=A  AffineConversion=off
  1 : PMIOPort  Port=1  Side=Left
  2 : PMIOPort  Port=2  Side=Right
  tag scope: I_ABC2=global
  wires:
  PS-Simulink Converter/1 -> [I_ABC2]
  connections:
  Current Sensor/RConn1 -- PS-Simulink Converter/LConn1
  2/RConn1 -- Current Sensor/RConn2
  1/RConn1 -- Current Sensor/LConn1

== system pe_electric_engine_dyno/Meas V ==
  PS-Simulink Converter4 : nesl_utility/PS-Simulink Converter  PhysicalDomain=network_engine_domain  SubClassName=ps_output  LeftPortType=input  RightPortType=output  PseudoPeriodic=off  Frequencies=[]  Unit=V  AffineConversion=off
  Voltage Sensor : fl_lib/Electrical/Electrical Sensors/Voltage Sensor
      settings: SourceProductName=Foundation Library
  + : PMIOPort  Port=1  Side=Left
  - : PMIOPort  Port=2  Side=Right
  tag scope: Vdc=global
  wires:
  PS-Simulink Converter4/1 -> [Vdc]
  connections:
  Voltage Sensor/LConn1 -- +/RConn1
  Voltage Sensor/RConn2 -- -/RConn1
  PS-Simulink Converter4/LConn1 -- Voltage Sensor/RConn1

== system pe_electric_engine_dyno/Meas V1 ==
  PS-Simulink Converter4 : nesl_utility/PS-Simulink Converter  PhysicalDomain=network_engine_domain  SubClassName=ps_output  LeftPortType=input  RightPortType=output  PseudoPeriodic=off  Frequencies=[]  Unit=V  AffineConversion=off
  Voltage Sensor : fl_lib/Electrical/Electrical Sensors/Voltage Sensor
      settings: SourceProductName=Foundation Library
  + : PMIOPort  Port=1  Side=Left
  - : PMIOPort  Port=2  Side=Right
  tag scope: Vdc2=global
  wires:
  PS-Simulink Converter4/1 -> [Vdc2]
  connections:
  PS-Simulink Converter4/LConn1 -- Voltage Sensor/RConn1
  Voltage Sensor/RConn2 -- -/RConn1
  Voltage Sensor/LConn1 -- +/RConn1

== system pe_electric_engine_dyno/Tq Request ==
  Demux : Demux  Tag=STV Demux  Outputs=1
  FromWs : FromWorkspace  Tag=STV FromWs  VariableName=tuvar  SampleTime=0
      SigBuilderData=|
      | common.afterFinalStr = 'Extrapolate'
      | common.sampleTime = 0
      | dataSet.timeRange = [0 0.8]
      | dataSet.name = 'Group 1'
      | sbobj.Groups.Name = 'Group 1'
      | sbobj.Groups.Signals.Name = 'TqRequest'
      | sbobj.Groups.Signals.XData = [0 0.11 0.11 0.23 0.23 0.318 0.318 0.42 0.42 0.565 0.565 0.704 0.704 0.8]
      | sbobj.Groups.Signals.YData = [0 0 100 100 150 150 205 205 60.5 60.5 -56 -56 -155 -155]
      | sbobj.Groups.TimeRange = [0 0.8]
  TqRequest : Outport  Tag=STV Outport
  wires:
  Demux/1 -> TqRequest/1
  FromWs/1 -> Demux/1

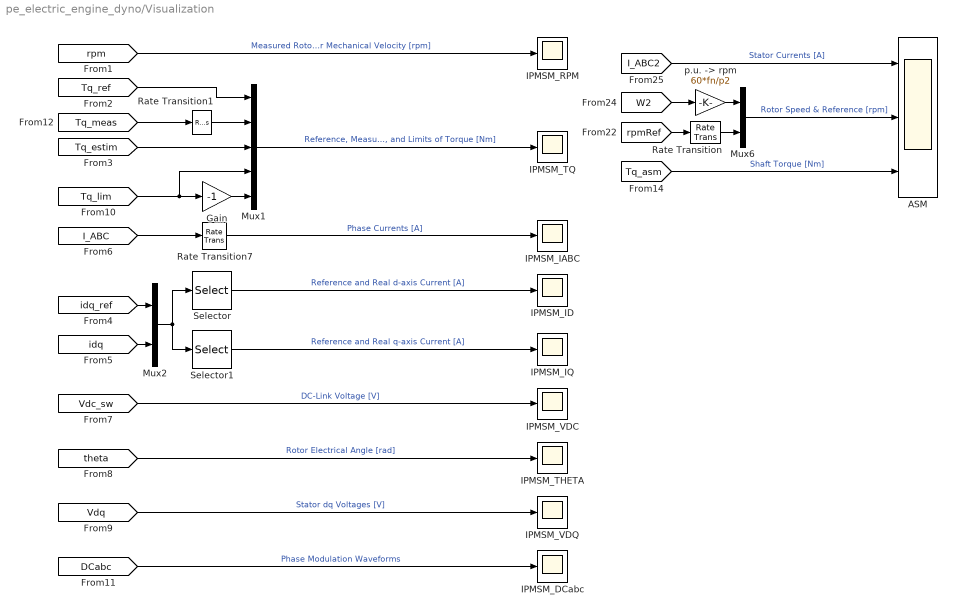
== system pe_electric_engine_dyno/Visualization ==
  ASM : Scope  NumInputPorts=3
  Gain : Gain  Gain=-1
  IPMSM_DCabc : Scope
  IPMSM_IABC : Scope
  IPMSM_ID : Scope
  IPMSM_IQ : Scope
  IPMSM_RPM : Scope
  IPMSM_THETA : Scope
  IPMSM_TQ : Scope
  IPMSM_VDC : Scope
  IPMSM_VDQ : Scope
  Mux1 : Mux  Inputs=5
  Mux2 : Mux  Inputs=2
  Mux6 : Mux  Inputs=2
  Rate Transition : RateTransition
  Rate Transition1 : RateTransition
  Rate Transition7 : RateTransition  OutPortSampleTime=1e-4
  Selector : Selector  InputPortWidth=4  IndexOptions=Index vector (dialog)  Indices=[1 3]  OutputSizes=1
  Selector1 : Selector  InputPortWidth=4  IndexOptions=Index vector (dialog)  Indices=[2 4]  OutputSizes=1
  "p.u. -> rpm" : Gain  Gain=60*fn/p2
  wires:
  [rpm] -> IPMSM_RPM/1  "Measured Rotor Mechanical Velocity [rpm]"
  Mux1/1 -> IPMSM_TQ/1  "Reference, Measured, Estim, and Limits of Torque [Nm]"
  [Tq_ref] -> Mux1/1
  [I_ABC] -> Rate Transition7/1
  [Vdc_sw] -> IPMSM_VDC/1  "DC-Link Voltage [V]"
  [theta] -> IPMSM_THETA/1  "Rotor Electrical Angle [rad]"
  [Vdq] -> IPMSM_VDQ/1  "Stator dq Voltages [V]"
  [Tq_lim] -> Mux1/4, Gain/1
  [DCabc] -> IPMSM_DCabc/1  "Phase Modulation Waveforms"
  [W2] -> "p.u. -> rpm"/1
  [I_ABC2] -> ASM/1  "Stator Currents [A]"
  Mux6/1 -> ASM/2  "Rotor Speed & Reference [rpm]"
  [rpmRef] -> Rate Transition/1
  "p.u. -> rpm"/1 -> Mux6/1
  Rate Transition/1 -> Mux6/2
  Rate Transition7/1 -> IPMSM_IABC/1  "Phase Currents [A]"
  Selector1/1 -> IPMSM_IQ/1  "Reference and Real q-axis Current [A]"
  [idq_ref] -> Mux2/1
  Selector/1 -> IPMSM_ID/1  "Reference and Real d-axis Current [A]"
  Mux2/1 -> Selector1/1, Selector/1
  [idq] -> Mux2/2
  [Tq_meas] -> Rate Transition1/1
  Gain/1 -> Mux1/5
  Rate Transition1/1 -> Mux1/2
  [Tq_estim] -> Mux1/3
  [Tq_asm] -> ASM/3  "Shaft Torque [Nm]"

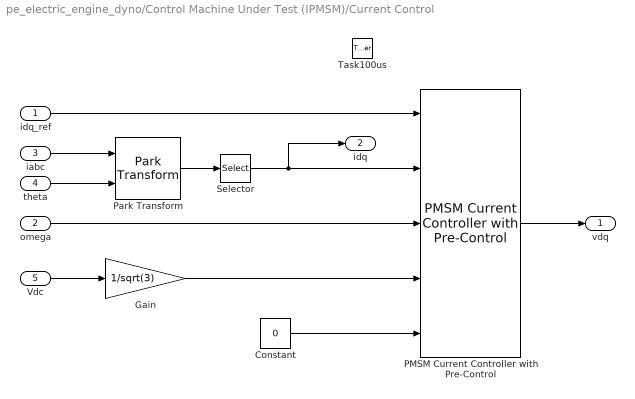
== system pe_electric_engine_dyno/Control Machine Under Test (IPMSM)/Current Control ==
  idq_ref : Inport
  omega : Inport  Port=2
  iabc : Inport  Port=3
  theta : Inport  Port=4
  Vdc : Inport  Port=5
  Task100us : TriggerPort  TriggerType=function-call  VariantControl=Variant  PortDimensions=1
  Constant : Constant  Value=0  SampleTime=-1
  Gain : Gain  Gain=1/sqrt(3)
  PMSM Current Controller with Pre-Control : pePmsmCurrentController/PMSM Current Controller with Pre-Control  Kp_id=Kp_id  Ki_id=Ki_id  Kaw_id=1  Kp_iq=Kp_iq  Ki_iq=Ki_iq  Kaw_iq=1  Ts=-1  Tsd=Tsi  AxisPrio=Q-axis  ActZC=on  ActFF=on  idVect=[-200, 0, 200]  iqVect=[-200, 0, 200]  LdMatrix=Ld * ones(3, 3)  LqMatrix=Lq * ones(3, 3)  psimMatrix=psim * ones(3, 3)
  Park Transform : peTransforms/Park Transform  AxisAlignment=Q-axis  PowerInvariant=off
  Selector : Selector  InputPortWidth=3  IndexOptions=Index vector (dialog)  Indices=[1 2]  OutputSizes=1
  vdq : Outport
  idq : Outport  Port=2
  wires:
  idq_ref/1 -> PMSM Current Controller with Pre-Control/1
  iabc/1 -> Park Transform/1
  theta/1 -> Park Transform/2
  omega/1 -> PMSM Current Controller with Pre-Control/3
  Vdc/1 -> Gain/1
  Gain/1 -> PMSM Current Controller with Pre-Control/4
  Constant/1 -> PMSM Current Controller with Pre-Control/5
  PMSM Current Controller with Pre-Control/1 -> vdq/1
  Selector/1 -> idq/1, PMSM Current Controller with Pre-Control/2
  Park Transform/1 -> Selector/1

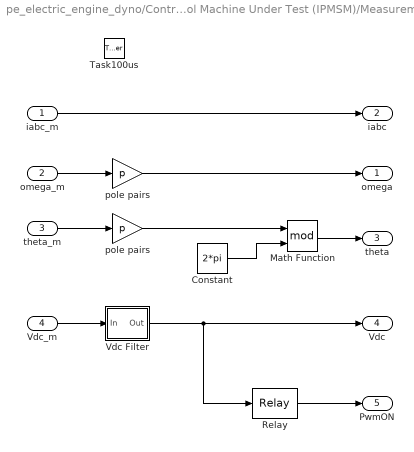
== system pe_electric_engine_dyno/Control Machine Under Test (IPMSM)/Measurements ==
  iabc_m : Inport
  omega_m : Inport  Port=2
  theta_m : Inport  Port=3
  Vdc_m : Inport  Port=4
  Task100us : TriggerPort  TriggerType=function-call  VariantControl=Variant  PortDimensions=1
  Constant : Constant  Value=2*pi  SampleTime=-1
  Math Function : Math  Operator=mod  SaturateOnIntegerOverflow=on
  Relay : Relay  OnSwitchValue=VDC_VECT(1)  OffSwitchValue=0.5*VDC_VECT(1)
  Vdc Filter : Subsystem  mask(Discrete first-order filter (Low-pass)){T=0.005, Ts=1e-4}
      mask prompts: T "Time constant (s):"; Ts "Sample time (s):"
      mask help: This block implements a discrete low-pass filter. To calculate the coefficients, the block discretises a continuous low-pass filter using the Tustin method.
      mask init:
      | num = [ Ts/(2*T + Ts), Ts/(2*T + Ts)];
      | den = [ 1, -(2*T - Ts)/(2*T + Ts)];
  pole pairs : Gain  Gain=p
  "pole pairs " : Gain  Gain=p
  omega : Outport
  iabc : Outport  Port=2
  theta : Outport  Port=3
  Vdc : Outport  Port=4
  PwmON : Outport  Port=5
  wires:
  pole pairs/1 -> omega/1
  theta_m/1 -> "pole pairs "/1
  omega_m/1 -> pole pairs/1
  iabc_m/1 -> iabc/1
  "pole pairs "/1 -> Math Function/1
  Constant/1 -> Math Function/2
  Math Function/1 -> theta/1
  Vdc_m/1 -> Vdc Filter/1(In)
  Relay/1 -> PwmON/1
  Vdc Filter/1(Out) -> Relay/1, Vdc/1

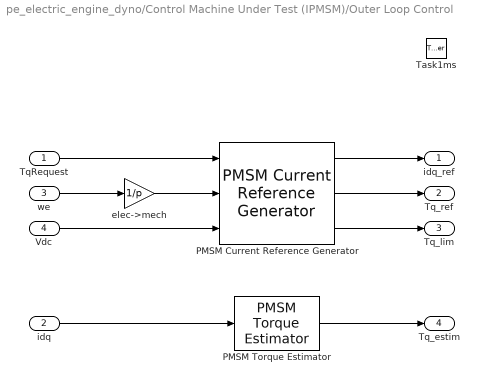
== system pe_electric_engine_dyno/Control Machine Under Test (IPMSM)/Outer Loop Control ==
  TqRequest : Inport
  idq : Inport  Port=2
  we : Inport  Port=3
  Vdc : Inport  Port=4
  Task1ms : TriggerPort  TriggerType=function-call  VariantControl=Variant  PortDimensions=1
  PMSM Current Reference Generator : pePmsmCurrentReferenceGen/PMSM Current Reference Generator  Vnom=Vnom  Pmax=Pmax  Tmax=Tmax  Ts=-1  RefType=Lookup-table based  rpmVec=RPM_VECT  TqVec=TQ_VECT  VdcVec=VDC_VECT  idMatrix=ID_MAP  iqMatrix=IQ_MAP  p=8  psim=0.04  Ld=0.00024  Lq=0.00029  Rs=0.01  RefExpEnable=0
  PMSM Torque Estimator : pePmsmTorqueEstimator/PMSM Torque Estimator  ParamType=Constant parameters  p=p  idVect=[-200, 200]  iqVect=[-200, 200]  LdMatrix=0.0002 * ones(2, 2)  LqMatrix=0.0002 * ones(2, 2)  psimMatrix=0.04 * ones(2, 2)  Ld=Ld  Lq=Lq  psim=psim  Ts=-1
  elec->mech : Gain  Gain=1/p
  idq_ref : Outport
  Tq_ref : Outport  Port=2
  Tq_lim : Outport  Port=3
  Tq_estim : Outport  Port=4
  wires:
  PMSM Current Reference Generator/1 -> idq_ref/1
  PMSM Torque Estimator/1 -> Tq_estim/1
  idq/1 -> PMSM Torque Estimator/1
  elec->mech/1 -> PMSM Current Reference Generator/2
  Vdc/1 -> PMSM Current Reference Generator/3
  PMSM Current Reference Generator/2 -> Tq_ref/1
  TqRequest/1 -> PMSM Current Reference Generator/1
  we/1 -> elec->mech/1
  PMSM Current Reference Generator/3 -> Tq_lim/1

== system pe_electric_engine_dyno/Control Machine Under Test (IPMSM)/Measurements/Vdc Filter ==
  In : Inport
  Discrete Transfer Fcn : DiscreteTransferFcn  Numerator=num  Denominator=den
  Out : Outport
  wires:
  Discrete Transfer Fcn/1 -> Out/1
  In/1 -> Discrete Transfer Fcn/1

== stateflow chart pe_electric_engine_dyno/Control Machine Under Test (IPMSM)/Task Scheduler ==
  (default) -> (junction 23) : CLK_50us
  (junction 23) -> (junction 17)
  (junction 17) -> (junction 22) [order 2]
  (junction 17) -> (junction 22) [order 1] : [cnt%%2==0]{Task_100us_1;}
  (junction 22) -> (junction 18) [order 2]
  (junction 22) -> (junction 18) [order 1] : [cnt%%2==0]{Task_100us_2;}
  (junction 18) -> (junction 21) [order 2]
  (junction 18) -> (junction 21) [order 1] : [cnt%%20==0]{Task_1ms_1;}
  (junction 21) -> (junction 34) [order 2]
  (junction 21) -> (junction 16) [order 1] : [1]{cnt++;}
  data: cnt local int32
  events: Task_100us_1 output FUNCTION_CALL_EVENT; Task_100us_2 output FUNCTION_CALL_EVENT; Task_1ms_1 output FUNCTION_CALL_EVENT; CLK_50us input FUNCTION_CALL_EVENT
